simulink model "theta_control"  (R2021a)
settings: Solver=VariableStepAuto  StartTime=0.0  StopTime=10  RelTol=1e-3
libraries: simulink x1
settings Model: Creator=JianFongLee  LastModifiedBy=JianFongLee
settings SolverCC: AlgebraicLoopSolver=TrustRegion
settings DebuggingCC: SFMachineParentedDataDiag=warning

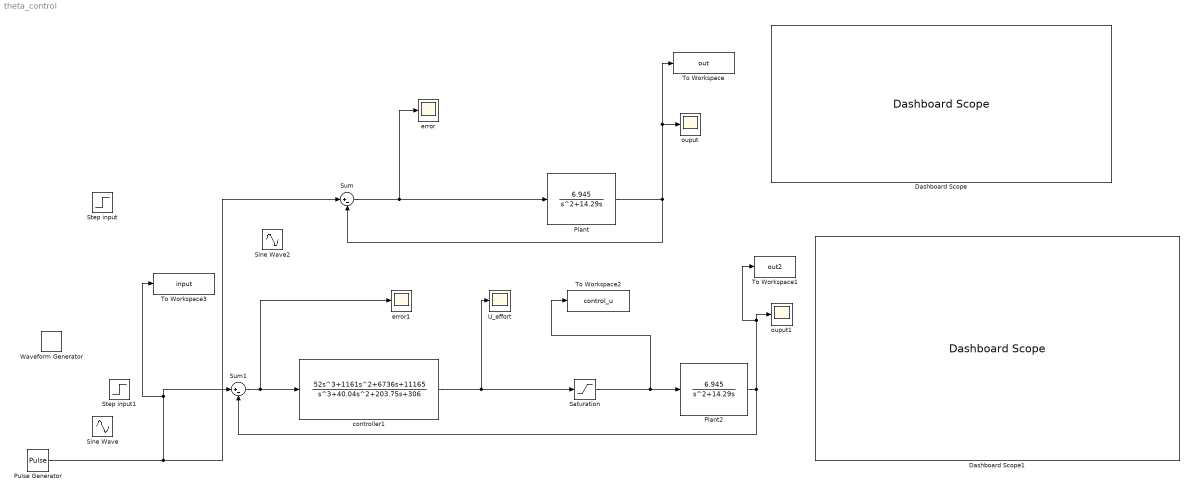
== system theta_control ==
  " Plant" : TransferFcn  Numerator=[6.945]  Denominator=[1 14.29 0]
  " Plant2" : TransferFcn  Numerator=[6.945]  Denominator=[1 14.29 0]
  Dashboard Scope : DashboardScope
  Dashboard Scope1 : DashboardScope
  Pulse Generator : DiscretePulseGenerator  PulseType=Time based  Period=20  PulseWidth=50
  Saturation : Saturate  UpperLimit=12  LowerLimit=-12
  Sine Wave : Sin  Frequency=5  Phase=20  SampleTime=0
  Sine Wave2 : Sin  Frequency=10  SampleTime=0
  Step input : Step  Time=0  SampleTime=0
  Step input1 : Step  Time=0  SampleTime=0
  Sum : Sum  Inputs=|+-
  Sum1 : Sum  Inputs=|+-
  To Workspace : ToWorkspace  VariableName=out  SaveFormat=Timeseries  SampleTime=-1
  To Workspace1 : ToWorkspace  VariableName=out2  SaveFormat=Timeseries  SampleTime=-1
  To Workspace2 : ToWorkspace  VariableName=control_u  SaveFormat=Timeseries  SampleTime=-1
  To Workspace3 : ToWorkspace  VariableName=input  SaveFormat=Timeseries  SampleTime=-1
  U_effort : Scope
  Waveform Generator : simulink/Sources/Waveform Generator  OutMin=[]  OutMax=[]  OutDataTypeStr=double  SelectedSignal=1  BlockNames=MultiportSwitch_e3df3653d217406  SampleTime=0.1
  controller1 : TransferFcn  Numerator=[52 1161 6736 11165]  Denominator=[1 40.04 203.75 306]
  error : Scope
  error1 : Scope
  ouput : Scope
  ouput1 : Scope
  wires:
  Sum/1 -> error/1, " Plant"/1
  " Plant"/1 -> Sum/2, To Workspace/1, ouput/1
  " Plant2"/1 -> Sum1/2, To Workspace1/1, ouput1/1
  Sum1/1 -> controller1/1, error1/1
  controller1/1 -> U_effort/1, Saturation/1
  Saturation/1 -> To Workspace2/1, " Plant2"/1
  Pulse Generator/1 -> Sum/1, To Workspace3/1, Sum1/1
